simulink model "F16ASYM_Controlled_AoA"  (R2012b)
settings: Solver=ode3  SolverMode=SingleTasking  StartTime=0.0  StopTime=inf  FixedStep=T_sim  RelTol=1e-3
InitFcn:
  | load('NN_c_weights_Last_stable.mat')
values from neighbouring files (symbols this model uses):
  K_b_AoA = params(3)    [Cost_function.m]
  K_b_q = params(4)    [Cost_function.m]
  learning = 20    [Scheduling_desing.m]
  Model_used_flag = 1    [Scheduling_desing.m]
  reg_param = 0.5    [Scheduling_desing.m]
  T_sim = 0.02    [Scheduling_desing.m]
  tau_AoA = params(1)    [Cost_function.m]
  tau_q = params(2)    [Cost_function.m]
  Theta_1_roll_last = [0.00183613313267 0.00115998993235 0.0006676025148 0.00194921904952 0.00134963559861 0.00034352059664 0.000447169388141 0.00146749660935 0.00110199952389 7.77922383894e-05 0.00109492833348 0.00192687590535 ... (360 elements, 30x12)]    [NN_i_weights_LAST_STABLE.mat]
  Theta_2_roll_last = [0.000469743069697 0.000355923851088 0.00180035760697 0.00191855117771 0.00118851504447 0.0013331642065 0.0013164316578 0.000643981263341 0.00176817665434 0.000113802099363 0.000426534542462 0.00113815782354 ... (620 elements, 20x31)]    [NN_i_weights_LAST_STABLE.mat]
  Theta_3_roll_last = [9.62071520568e-05 -0.000389870886846 2.08260845013e-05 0.000140787743673 -0.000917525755397 -0.0014324207578 -0.00154701573815 -0.00131544476264 -0.00101205584381 5.06515794689e-05 -0.00111443483676 -0.00143957416141 ... (21 elements, 1x21)]    [NN_i_weights_LAST_STABLE.mat]
  V_long_lastA_w_z = [0.352826086601 -0.253633004548 -0.642535042878 0.237749930435 -0.618390629538 0.858074761295 0.268211230628 -0.448715080196 -0.0406384631192 0.401147605577 0.60598427709 0.0500551915851 ... (300 elements, 30x10)]    [NN_i_weights_LAST_STABLE.mat]
  V_long_lastAoA = [0.0774300162379 0.0911421319631 0.0352371192557 0.0542170286952 0.0651171200844 0.0177112012707 0.0982957728448 0.000259994642558 0.0194724569123 0.0466321328252 0.0556687953852 0.0252668067142 ... (300 elements, 30x10)]    [NN_i_weights_LAST_STABLE.mat]
  V_roll_last = [0.0540918675943 0.0557493347212 0.0839792276608 0.0460576391794 0.0671229058124 0.100220403067 0.0722493281881 0.0648875457457 0.00447599349201 0.0607299103823 0.0488037966361 0.0176785979393 ... (360 elements, 30x12)]    [NN_i_weights_LAST_STABLE.mat]
  V_yaw_last = [0.0965149149679 0.00833616709545 0.0365734360076 0.0523944217566 0.00790252078455 0.0700053845887 0.0345164868709 0.0111568465295 0.094060639546 0.0205483560006 0.000798047494256 0.0862769385758 ... (360 elements, 30x12)]    [NN_i_weights_LAST_STABLE.mat]
  velocity = M_eval_sche(I,J)*a    [Scheduling_desing.m]
  W_long_lastA_w_z = [-0.0522913429974 0.00385484301394 -0.00465489482472 -0.0139416219936 0.00295196421483 -0.013027768541 0.00585545058915 0.00278802233571 -0.00906272782329 -0.000396112031465 0.00405849743321 0.00509668457818 ... (31 elements, 1x31)]    [NN_i_weights_LAST_STABLE.mat]
  W_long_lastAoA = [-0.0192589013922 0.00873109909713 0.00432649597332 0.0420946902441 0.0293366820194 0.0351497798191 0.0234952374236 0.0360841187718 0.0112233388211 0.030147202199 0.0369533138617 0.00218839076415 ... (31 elements, 1x31)]    [NN_i_weights_LAST_STABLE.mat]
  W_roll_last = [-0.0006515532842 0.000535485585715 0.000550946920743 0.000806030945453 0.00045976209382 0.00065557954304 0.000945902185602 0.00070191398535 0.000635215543728 4.66501377412e-05 0.000597079583757 0.000485790566765 ... (31 elements, 1x31)]    [NN_i_weights_LAST_STABLE.mat]
  W_yaw_last = [-4.34263633305e-05 8.83823048922e-05 1.65575463724e-05 3.60293102233e-05 5.19752447623e-05 7.06399280852e-06 7.02425975821e-05 3.62680255076e-05 1.29996379937e-05 8.05072914397e-05 2.39941870661e-05 2.52427840574e-06 ... (31 elements, 1x31)]    [NN_i_weights_LAST_STABLE.mat]
undefined symbols (not defined in the file or in its folder): a1, alpha_map_eval, B, beta_map_eval, C_L_0, DiscIntNeverNeededParam, fi_flag_Simulink, G_eval, H_sq, H_sq_autotrim, k_B, m_B, M_sq, M_sq_autotrim, sigbuilder_block, Stall_curve, trim_control, trim_state, trim_throttle, V_Comp_A_w_z_last, V_Comp_last, V_roll_lastMOD, W_Comp_A_w_z_last, W_Comp_last, W_roll_lastMOD
libraries: Adaptive_FaultTolerantControl x43, dspsigops x29, F16_Actuator_Library x14, simulink x8, aerolibatmos2 x7, dsparch4 x6, simulink_extras x5, aerolibtransform2 x5, qcatlib x4, dspmtrx3 x3, dspvision x2, dspsnks4 x2
(part 9 of 11)

== matlab function F16ASYM_Controlled_AoA/SI and FDI/SI and FDI: Realistic/SI/Surfaces UKF estimator ==
  data: P input; P_out output; X_ant input; Meas input; Alt input; S_l output; TAS input; AoA input; SS input; omega_b input; Control_def input; Ctrl_effectiveness input; Deltas_Aero input; S_r output; S_f output
function [P_out,S_l,S_r,S_f] = UKF_estimator(P,X_ant,Meas,Alt,TAS,AoA,SS,omega_b,Control_def,Ctrl_effectiveness,Deltas_Aero)
% Control_def includes Throttle
% Meas are angular accelerations

m = 9295.44;
x_cg = 0.3;
Jy=75673.6;
Jxz=1331.4;
Jz=85552.1;
Jx=12874.8;

Ang_accels = zeros(3,1);
coder.extrinsic('Ang_accels_Reconf_estimator');
coder.extrinsic('schol');
coder.extrinsic('chol');

% Ang_accels = Ang_accels_Reconf_estimator([Alt,TAS,AoA,SS,omega_b',Control_def',m,  X_ant'  ,x_cg,Jy,Jxz,Jz,Jx,Ctrl_effectiveness',Deltas_Aero']');
% Ang_accels
% C_l = Ang_accels(1)
% C_m = Ang_accels(2)
% C_n = Ang_accels(3)


% S_l = 27.87/2;
% S_r=S_l;
% S_f = 6.578;
% P_out = P;


%% Filter UKF
% Init parameters 
F = eye(3);
Q = 0.005*eye(3); % Noise in the process (in surfaces)
R = 20*eye(3);   % Noise in the measures of angular acceleration

% Prediction . IT is a simple linear prediction. There is not need to do it
% in any other way because the result is the SAME
    x_pred=F*X_ant;
    x_pred(1) = max(0,min(x_pred(1),27.87/2));
    x_pred(2) = max(0,min(x_pred(2),27.87/2));
    x_pred(3) = max(0,min(x_pred(3),6.578));

    P_pred = F * P * F' + Q;

% Uncested Update
    % Measurement equations.
%     Ang_accels_Reconf_estimator([Alt,TAS,AoA,SS,omega_b',Control_def',m,  X_ant'  ,x_cg,Jy,Jxz,Jz,Jx,Ctrl_effectiveness',Deltas_Aero']')

    % Weight params
    L=size(X_ant,1);
    alpha = 1;  beta = 0;   kappa = 3 - L; % Supposed as optimals
    % %                 alpha = 0.6;  beta = 1.3;   kappa = 0.9; % Optimized by me
    
    % Generate_weights
        W_s = zeros(2*L+1,1);
        W_c = zeros(2*L+1,1);
        lambda = alpha^2 * (L + kappa) - L;
        for j=1:2*L+1
            if j==1
                W_s(j) = lambda / (L + lambda);
                W_c(j) = lambda / (L + lambda) + (1 - alpha^2 + beta);
            else
                W_s(j) = 1 / (2 * (L + lambda));
                W_c(j) = W_s(j);
            end
        end
        
    % Sigma_points
            flag = 0;
            A = zeros(size(P));
            [A,flag] = chol(P);
            A = A';
            if flag>0
                A = schol(P);
            end
        X = [zeros(size(x_pred)) A -A];
        X = sqrt(L + lambda)*X + repmat(x_pred,1,size(X,2));

    % Propagation with measurement equation (Model in this case)
        gamma_z = zeros(3,size(X,2));
        gamma_z(:,1) = Ang_accels_Reconf_estimator([Alt,TAS,AoA,SS,omega_b',Control_def',m,  X(:,1)'  ,x_cg,Jy,Jxz,Jz,Jx,Ctrl_effectiveness',Deltas_Aero']');
        for i=2:size(X,2)
%             [Alt,TAS,alpha,beta,omega_b',Control_def',m,  X(:,1)'  ,x_cg,Jy,Jxz,Jz,Jx,Ctrl_effectiveness',Deltas_Aero']
            gamma_z(:,i) = Ang_accels_Reconf_estimator([Alt,TAS,AoA,SS,omega_b',Control_def',m,  X(:,i)'  ,x_cg,Jy,Jxz,Jz,Jx,Ctrl_effectiveness',Deltas_Aero']');
        end
        
    % Update
    Z = zeros(size(gamma_z,1),1);
    Pzz  = zeros(size(gamma_z,1),size(gamma_z,1));
    Pxz  = zeros(size(x_pred,1),size(gamma_z,1));
    for i=1:size(X,2)
        Z = Z + W_s(i) * gamma_z(:,i);
    end
    for i=1:size(X,2)
        Pzz = Pzz + W_c(i) * (gamma_z(:,i) - Z) * (gamma_z(:,i) - Z)';
        Pxz = Pxz + W_c(i) * (X(1:size(x_pred,1),i) - x_pred) * (gamma_z(:,i) - Z)';
    end

    Pzz = Pzz + R;
    K = Pxz / Pzz;
    x_estimate = x_pred + K * (Meas - Z);
    P_out = P_pred - K * Pzz * K';
%     x_estimate
    S_l = x_estimate(1);
    S_r = x_estimate(2);
    S_f = x_estimate(3);

== matlab function F16ASYM_Controlled_AoA/Primary Controller/P  + Crossed NN + AWU+Lim + hand-over/P controller + adaptive Crossed NN + AWU+Lim    in ACC /Complete crossed On-line (adaptive) multi-layer NN: A_w_z/Cross NN A_w_z ==
  data: X_bar input size=[25,1]; v_ad_comp output; e input; Factor_F input; K_roll input; Ks_long input; Ks_yaw input; B input; Learnign_rate input size=1; Reg_param input size=1; AWU input; W input size=[3,51]; V input size=[50,25]; v_ad output; Z_norm_unit output; T_sim parameter; W_update output; V_update output
function [v_ad_comp,v_ad,Z_norm_unit,W_update,V_update]  = Cross_NN(X_bar,e,Factor_F, K_roll,Ks_long,Ks_yaw,B,Learnign_rate,Reg_param,AWU,W,V,T_sim)

%% Compute prelimiary parametes
% Compute P with regular Lyapunov equation solution
P_roll=1/K_roll;
P_long =  [   1/Ks_long(1) , Factor_F/(Ks_long(1)^2+Ks_long(1)*Ks_long(2));
     1/(Ks_long(1)^2+Ks_long(1)*Ks_long(2)) ,(Ks_long(1)^2+Ks_long(1)*Ks_long(2)+Factor_F^2)/(Ks_long(2)^2*Ks_long(1)+Ks_long(2)*Ks_long(1)^2) ];
P_yaw = [   1/Ks_yaw(1) , 1/(Ks_yaw(1)^2+Ks_yaw(1)*Ks_yaw(2));
     1/(Ks_yaw(1)^2+Ks_yaw(1)*Ks_yaw(2)) ,(Ks_yaw(1)^2+Ks_yaw(1)*Ks_yaw(2)+1)/(Ks_yaw(2)^2*Ks_yaw(1)+Ks_yaw(2)*Ks_yaw(1)^2) ];
 
P = blkdiag(P_roll,P_long,P_yaw);

% % % % Compute P with on-line Lyapunov equation solution
% % % CROSS = 0;
% % % A = [ -K_roll,0,CROSS,0,0;0,-Ks_long(1),1,0,0;
% % %     0,0,-Ks_long(2),0,0;0,0,0,-Ks_yaw(1),Factor_F;0,0,0,0,-Ks_yaw(2)];
% % % 
% % % coder.extrinsic('lyap')
% % % P = A;
% % % P = lyap(A,2*diag(ones(5,1)));



K_awu = 1.2;
zeta= e'*P*B;


% Introduce Anti-windup
zeta = zeta - K_awu*AWU'.*T_sim; 

% Convergence limitation
if norm(zeta)>2/(T_sim*Learnign_rate*Reg_param)
    zeta = (zeta./norm(zeta)).*(1.8/(T_sim*Learnign_rate*Reg_param));
end

%% Feedforward
z = V*X_bar;
s=sigmoid(V*X_bar);

sigma = [1 ; s ];
% v_ad = W*sigma;

sigma_grad = (sigma.*(ones(size(sigma))-sigma));

%% Compute the gradients or adaptation laws
Gamma_w= Learnign_rate; % W learnign rate
Gamma_v= Learnign_rate; %V learning rate
lambda = Reg_param;

V_dot=zeros(size(V));
W_dot=zeros(size(W));

W_dot= -Gamma_w*(  (sigma - sigma_grad.*[1;z] )*zeta  )';
W_dot(:,2:end)= W_dot(:,2:end) - Gamma_w*lambda*norm(zeta)*(W(:,2:end));

M = W'*zeta'.*sigma_grad ;
V_dot= -Gamma_v*( M(2:end)*X_bar'  );
V_dot(:,2:end)= V_dot(:,2:end) - Gamma_v*lambda*norm(zeta).*V(:,2:end);

% % % Other way: Based on notes of Andrew NG
% % 
% % delta2=W'*zeta'.*sigma_grad;
% % 
% % V_dot = - Gamma_v*( delta2(2:end)*X_bar');
% % V_dot(:,2:end)= V_dot(:,2:end) - Gamma_v*lambda*norm(zeta).*V(:,2:end);
% % 
% % W_dot = - Gamma_w*( sigma*zeta)';
% % W_dot(:,2:end)= W_dot(:,2:end) - Gamma_w*lambda*norm(zeta)*(W(:,2:end));



%% Adaptation
W_update = W + T_sim*W_dot;
V_update = V + T_sim*V_dot;
% 
%% Re-compute v_ad

s=sigmoid(V_update*X_bar);

sigma = [1 ; s(:,1) ];
v_ad = W_update*sigma;

%% Compute v_ad_comp
Z = [ V,zeros(size(V,1),size(W,2));
    zeros(size(W,1),size(V,2)),W];
    
Z_norm = norm(Z,'fro');
Z_max = 2*min(size(W,1),size(W,2) )*min( size(V,1),size(V,2) );
Z_norm_unit = Z_norm;

K_r0= 0;
K_r1= 0;
v_r0 = -K_r0*zeta';
v_r1 = -K_r1*(Z_norm+Z_max)*zeta';

v_ad_comp = v_ad + v_r1 +v_r0;

% % % Normalization of matrices
% % if Z_norm>Z_max
% %     V = (V.*Z_max)./Z_norm;
% %     W = (W.*Z_max)./Z_norm;
% % end
end

== system F16ASYM_Controlled_AoA/Primary Controller/P controller + adaptive Crossed NN + AWU+Lim /Complete crossed On-line (adaptive) multi-layer NN/Complete crossed On-line (adaptive) multi-layer NN: AoA ==
  v_ad^ prev : Inport
  All_meas : Inport  Port=2
  NN variables : Inport  Port=3
  AWU : Inport  Port=4
  B : Constant  Value=[1 0 0;0 0 0;0 1 0;0 0 0;0 0 1]
  Bus Selector : BusSelector  OutputSignals=p_chanel_vars,Long chanel,beta_r_chanel
  Bus Selector1 : BusSelector  OutputSignals=p_err,p_sf,p_sf_dot,K_b_p
  Bus Selector2 : BusSelector  OutputSignals=signal1.Alt meas (m),signal2.Mach,signal1.AoA meas (rad),signal1.SS meas (rad),signal1.omega_b meas (rad/s)
  Bus Selector3 : BusSelector  OutputSignals=alpha_chanel vars.alpha_err,q_chanel_vars.q_err,alpha_chanel vars.alpha_sf,alpha_chanel vars.alpha_sf_dot,q_chanel_vars.q_sf_dot,alpha_chanel vars.K_b_alpha,q_chanel_vars.K_b_q
  Bus Selector4 : BusSelector  OutputSignals=beta_chanel vars.beta_err,r_chanel vars.r_err,beta_chanel vars.beta_sf,beta_chanel vars.beta_sf_dot,r_chanel vars.r_sf_dot,beta_chanel vars.K_b_beta,r_chanel vars.K_b_r
  C Learning rate : Constant  Value=30  SampleTime=T_sim
  C Reg param : Constant  Value=0.5  SampleTime=T_sim
  Constant : Constant
  Cross NN : MATLAB Function  TreatAsAtomicUnit=on
  Display : Display
  Divide : Product  Inputs=**
  Divide1 : Product  Inputs=**
  Memory2 : Memory  X0=V_Comp_last
  Memory3 : Memory  X0=W_Comp_last
  Mux1 : Mux  Inputs=9
  Mux10 : Mux  Inputs=3
  Mux2 : Mux  Inputs=3
  Mux{3..4,6..7} (4 alike) : Mux  Inputs=2
  Mux5 : Mux  Inputs=5
  Mux8 : Mux  Inputs=5
  Mux9 : Mux  Inputs=[9 3 5 5 3]
  Scope : Scope
      settings: SaveName=ScopeData8
  Selector : Selector  InputPortWidth=3  IndexOptions=Index vector (dialog)  Indices=1  OutputSizes=1
  Selector1 : Selector  InputPortWidth=3  IndexOptions=Index vector (dialog)  Indices=3  OutputSizes=1
  Terminator : Terminator
  Terminator1 : Terminator
  To Workspace : ToWorkspace  VariableName=V_Comp_last  SampleTime=-1
      settings: MaxDataPoints=1
  To Workspace1 : ToWorkspace  VariableName=W_Comp_last  SampleTime=-1
      settings: MaxDataPoints=1
  dem-less : Gain  Gain=T_sim
  dem-less1 : Gain  Gain=T_sim
  dem-less2 : Gain  Gain=T_sim^2
  dem-less3 : Gain  Gain=T_sim
  dem-less4 : Gain  Gain=T_sim^2
  dim-less : Gain  Gain=1/15000
  v_ad^ : Outport
  wires:
  Bus Selector/3 -> Bus Selector4/1  "<beta_r_chanel>"
  Bus Selector/2 -> Bus Selector3/1  "<Long chanel>"
  Bus Selector/1 -> Bus Selector1/1  "<p_chanel_vars>"
  NN variables/1 -> Bus Selector/1
  Bus Selector2/5 -> Selector1/1, Selector/1  "<omega_b meas (rad/s)>"
  dim-less/1 -> Mux1/2
  Divide1/1 -> Mux1/6
  Divide/1 -> Mux1/4
  Bus Selector2/1 -> dim-less/1  "<Alt meas (m)>"
  All_meas/1 -> Bus Selector2/1
  Constant/1 -> Mux1/1
  Bus Selector1/3 -> dem-less/1  "<p_sf_dot>"
  Selector/1 -> Mux1/8
  Bus Selector2/4 -> Mux1/7  "<SS meas (rad)>"
  Bus Selector2/2 -> Divide/2, Mux1/3, Divide/1  "<Mach>"
  Bus Selector2/3 -> Divide1/1, Mux1/5, Divide1/2  "<AoA meas (rad)>"
  Bus Selector1/4 -> [K_roll]  "<K_b_p>"
  Bus Selector1/2 -> Mux2/2  "<p_sf>"
  Bus Selector1/1 -> [e_roll], Mux2/1  "<p_err>"
  dem-less/1 -> Mux2/3
  dem-less2/1 -> Mux5/5
  dem-less1/1 -> Mux5/4
  Mux4/1 -> [Ks_long]
  Bus Selector3/6 -> Mux4/1  "<K_b_alpha>"
  Bus Selector3/7 -> Mux4/2  "<K_b_q>"
  Bus Selector3/5 -> dem-less2/1  "<q_sf_dot>"
  Bus Selector3/4 -> dem-less1/1  "<alpha_sf_dot>"
  Bus Selector3/1 -> Mux5/1, Mux3/1  "<alpha_err>"
  Bus Selector3/2 -> Mux5/2, Mux3/2  "<q_err>"
  Bus Selector3/3 -> Mux5/3  "<alpha_sf>"
  Mux3/1 -> [e_long]  "e"
  dem-less3/1 -> Mux8/4
  Bus Selector4/3 -> Mux8/3  "<beta_sf>"
  Bus Selector4/4 -> dem-less3/1  "<beta_sf_dot>"
  Bus Selector4/5 -> dem-less4/1  "<r_sf_dot>"
  Bus Selector4/7 -> Mux6/2  "<K_b_r>"
  Bus Selector4/6 -> Mux6/1  "<K_b_beta>"
  Mux6/1 -> [Ks_yaw]
  Bus Selector4/1 -> Mux8/1, Mux7/1  "<beta_err>"
  Bus Selector4/2 -> Mux8/2, Mux7/2  "<r_err>"
  Mux7/1 -> [e_yaw]  "e"
  dem-less4/1 -> Mux8/5
  Mux1/1 -> Mux9/1
  Mux2/1 -> Mux9/2
  Mux5/1 -> Mux9/3
  Mux8/1 -> Mux9/4
  v_ad^ prev/1 -> Mux9/5
  Mux9/1 -> Scope/1, Display/1, Cross NN/1(X_bar)
  Cross NN/3(Z_norm_unit) -> Terminator1/1
  C Reg param/1 -> Cross NN/8(Reg_param)
  C Learning rate/1 -> Cross NN/7(Learnign_rate)
  Cross NN/1(v_ad_comp) -> v_ad^/1
  Memory2/1 -> Cross NN/11(V)
  Memory3/1 -> Cross NN/10(W)
  B/1 -> Cross NN/6(B)
  Cross NN/2(v_ad) -> Terminator/1
  Cross NN/5(V_update) -> To Workspace/1, Memory2/1
  Cross NN/4(W_update) -> Memory3/1, To Workspace1/1
  Mux10/1 -> Cross NN/2(e)
  [e_roll] -> Mux10/1
  [e_long] -> Mux10/2
  [e_yaw] -> Mux10/3
  [K_roll] -> Cross NN/3(K_roll)
  [Ks_long] -> Cross NN/4(Ks_long)
  [Ks_yaw] -> Cross NN/5(Ks_yaw)
  Selector1/1 -> Mux1/9
  AWU/1 -> Cross NN/9(AWU)

== system F16ASYM_Controlled_AoA/Primary Controller/P controller + adaptive Crossed NN + AWU+Lim /Long Dyn Inversion: alpha_dot ->q/Completed ==
  alpha_dot_c : Inport
  All_meas : Inport  Port=2
  A_w_z : Selector  InputPortWidth=3  IndexOptions=Index vector (dialog)  Indices=3  OutputSizes=1
  Add : Sum
  Bus Selector : BusSelector  OutputSignals=signal1.AoA meas (rad),signal1.omega_b meas (rad/s),signal1.SS meas (rad),signal1.V_TAS (m/s),signal2.A_w_CG
  Display : Display
  Display1 : Display
  Display2 : Display
  Divide{,1..3} (4 alike) : Product  Inputs=**
  Divide4 : Product  Inputs=/*
  Selector : Selector  InputPortWidth=3  IndexOptions=Index vector (dialog)  Indices=1  OutputSizes=1
  Selector1 : Selector  InputPortWidth=3  IndexOptions=Index vector (dialog)  Indices=3  OutputSizes=1
  Trigonometric Function : Trigonometry  Operator=sincos
  Trigonometric Function1 : Trigonometry  Operator=tan
  Trigonometric Function2 : Trigonometry  Operator=cos
  "q_c " : Sum  Inputs=++-
  q_c : Outport
  wires:
  Trigonometric Function/1 -> Divide1/1
  Bus Selector/1 -> Trigonometric Function/1  "<AoA meas (rad)>"
  Selector/1 -> Divide/2
  Bus Selector/2 -> Selector1/1, Selector/1  "<omega_b meas (rad/s)>"
  Divide2/1 -> "q_c "/2, Display1/1
  Selector1/1 -> Divide1/2
  Divide3/1 -> Divide4/1
  alpha_dot_c/1 -> "q_c "/1, Display/1
  All_meas/1 -> Bus Selector/1
  Bus Selector/5 -> A_w_z/1  "<A_w_CG>"
  Bus Selector/3 -> Trigonometric Function1/1, Trigonometric Function2/1  "<SS meas (rad)>"
  Divide4/1 -> "q_c "/3
  "q_c "/1 -> q_c/1
  Divide/1 -> Add/1
  Bus Selector/4 -> Divide3/2  "<V_TAS (m/s)>"
  Add/1 -> Divide2/1
  Trigonometric Function1/1 -> Divide2/2
  Divide1/1 -> Add/2
  Trigonometric Function2/1 -> Divide3/1
  Trigonometric Function/2 -> Divide/1
  A_w_z/1 -> Display2/1, Divide4/2

== system F16ASYM_Controlled_AoA/Primary Controller/P controller + adaptive Crossed NN + AWU+Lim /Long Dyn Inversion: alpha_dot ->q/Simplified ==
  alpha_dot_c : Inport
  All_meas : Inport  Port=2
  A_b_z : Selector  InputPortWidth=3  IndexOptions=Index vector (dialog)  Indices=3  OutputSizes=1
  Bus Selector : BusSelector  OutputSignals=signal2.A_b_CG,signal1.V_TAS (m/s)
  Display : Display
  Divide4 : Product  Inputs=*/
  "q_c " : Sum  Inputs=+-
  q_c : Outport
  wires:
  "q_c "/1 -> q_c/1
  All_meas/1 -> Bus Selector/1
  alpha_dot_c/1 -> "q_c "/1, Display/1
  Bus Selector/2 -> Divide4/2  "<V_TAS (m/s)>"
  Divide4/1 -> "q_c "/2
  A_b_z/1 -> Divide4/1  "A_b_z"
  Bus Selector/1 -> A_b_z/1  "<A_b_CG>"

== system F16ASYM_Controlled_AoA/Primary Controller/P controller + adaptive Crossed NN + AWU+Lim /Longitudinal Controller: AoA or A_w_z/Longitudinal controller in A_w_z ==
  A_w_z des : Inport
  AoA des (rad) : Inport  Port=2
  Anti-windup A_w_z : Inport  Port=3
  Anti-windup AoA : Inport  Port=4
  All meas : Inport  Port=5
  Accel rate --> AoA rate! : Subsystem
  Bus Creator : BusCreator  Inputs=5
  Bus Selector : BusSelector  OutputSignals=signal2.A_w_CG
  Divide : Product  Inputs=**
  Gain : Gain  Gain=-1
  Ground : Ground
  Ref Model and P Controller : Adaptive_FaultTolerantControl/Ref Model and P Controller  tau=0.3  y_i=0  K_f=1  K_b=2.5
  Selector : Selector  InputPortWidth=3  IndexOptions=Index vector (dialog)  Indices=3  OutputSizes=1
  Stall protection : Subsystem  Commented=on
  Sum : Sum  Inputs=+-|
  Terminator : Terminator
  Terminator1 : Terminator
  Terminator2 : Terminator
  A_chanel vars : Outport
  alpha_chanel vars : Outport  Port=2
  alpha_dot_c : Outport  Port=3
  wires:
  Anti-windup AoA/1 -> Terminator1/1
  AoA des (rad)/1 -> Terminator/1
  Selector/1 -> Gain/1
  Gain/1 -> Ref Model and P Controller/2
  Bus Selector/1 -> Selector/1  "<A_w_CG>"
  Anti-windup A_w_z/1 -> Terminator2/1
  A_w_z des/1 -> Ref Model and P Controller/1
  Ref Model and P Controller/1 -> Divide/1
  Ref Model and P Controller/2 -> Bus Creator/1  "A_sf_dot"
  Ref Model and P Controller/3 -> Bus Creator/2, Sum/1  "A_sf"
  Sum/1 -> Bus Creator/3  "A_err"
  Ref Model and P Controller/4 -> Sum/2
  Ref Model and P Controller/5 -> Bus Creator/4  "K_b_A"
  Bus Creator/1 -> A_chanel vars/1
  Ground/1 -> alpha_chanel vars/1
  Divide/1 -> alpha_dot_c/1
  Accel rate --> AoA rate!/1(A_w  to AoA rates factor) -> Bus Creator/5, Divide/2  "FactorF"
  All meas/1 -> Bus Selector/1, Stall protection/2(All meas), Accel rate --> AoA rate!/1(All_meas)

== system F16ASYM_Controlled_AoA/Primary Controller/P controller + adaptive Crossed NN + AWU+Lim /Longitudinal Controller: AoA or A_w_z/Longitudinal controller in AoA ==
  A_w_z des : Inport
  AoA des (rad) : Inport  Port=2
  Anti-windup A_w_z : Inport  Port=3
  Anti-windup AoA : Inport  Port=4
  All meas : Inport  Port=5
  Bus Creator : BusCreator
  Bus Selector : BusSelector  OutputSignals=signal1.AoA meas (rad)
  Ground : Ground
  Ref Model and P Controller : Adaptive_FaultTolerantControl/Ref Model and P Controller  tau=0.3  y_i=trim_state(8)  K_f=1  K_b=8
  Sum : Sum  Inputs=+-|
  Terminator : Terminator
  Terminator1 : Terminator
  Terminator2 : Terminator
  A_chanel vars : Outport
  alpha_chanel vars : Outport  Port=2
  alpha_dot_c : Outport  Port=3
  wires:
  All meas/1 -> Bus Selector/1
  Ref Model and P Controller/1 -> alpha_dot_c/1
  Bus Selector/1 -> Ref Model and P Controller/2  "<AoA meas (rad)>"
  AoA des (rad)/1 -> Ref Model and P Controller/1
  A_w_z des/1 -> Terminator/1
  Anti-windup A_w_z/1 -> Terminator1/1
  Anti-windup AoA/1 -> Terminator2/1
  Ref Model and P Controller/2 -> Bus Creator/1  "alpha_sf_dot"
  Ref Model and P Controller/3 -> Sum/1, Bus Creator/2  "alpha_sf"
  Sum/1 -> Bus Creator/3  "alpha_err"
  Bus Creator/1 -> alpha_chanel vars/1
  Ref Model and P Controller/4 -> Sum/2
  Ref Model and P Controller/5 -> Bus Creator/4  "K_b_alpha"
  Ground/1 -> A_chanel vars/1

== system F16ASYM_Controlled_AoA/Primary Controller/P controller + adaptive Crossed NN + AWU+Lim /Physical limitation/Moments ==
  C_L : Inport
  C_M : Inport  Port=2
  C_N : Inport  Port=3
  q : Inport  Port=4
  B span : Constant  Value=9.144
  CMA : Constant  Value=3.45
  Divide : Product  Inputs=**
  Divide1 : Product  Inputs=***
  Divide2 : Product  Inputs=**
  Divide3 : Product  Inputs=***
  Divide4 : Product  Inputs=**
  S_w : Constant  Value=27.87
  S_w1 : Constant  Value=27.87
  q1 : InportShadow  Port=4
  L : Outport
  M : Outport  Port=2
  N : Outport  Port=3
  wires:
  Divide4/1 -> M/1  "M"
  Divide3/1 -> Divide4/2
  C_M/1 -> Divide4/1
  CMA/1 -> Divide3/3
  S_w1/1 -> Divide3/2
  q1/1 -> Divide3/1
  Divide2/1 -> N/1  "N"
  C_N/1 -> Divide2/2
  Divide/1 -> L/1  "L"
  Divide1/1 -> Divide/2, Divide2/1
  C_L/1 -> Divide/1
  B span/1 -> Divide1/3
  S_w/1 -> Divide1/2
  q/1 -> Divide1/1

== system F16ASYM_Controlled_AoA/Primary Controller/P controller + adaptive Isolated NN/Long Dyn Inversion: alpha_dot ->q/Completed ==
  alpha_dot_c : Inport
  All_meas : Inport  Port=2
  A_w_z : Selector  InputPortWidth=3  IndexOptions=Index vector (dialog)  Indices=3  OutputSizes=1
  Add : Sum
  Bus Selector : BusSelector  OutputSignals=signal1.AoA meas (rad),signal1.omega_b meas (rad/s),signal1.SS meas (rad),signal1.V_TAS (m/s),signal2.A_w_CG
  Display : Display
  Display1 : Display
  Display2 : Display
  Divide{,1..3} (4 alike) : Product  Inputs=**
  Divide4 : Product  Inputs=/*
  Selector : Selector  InputPortWidth=3  IndexOptions=Index vector (dialog)  Indices=1  OutputSizes=1
  Selector1 : Selector  InputPortWidth=3  IndexOptions=Index vector (dialog)  Indices=3  OutputSizes=1
  Trigonometric Function : Trigonometry  Operator=sincos
  Trigonometric Function1 : Trigonometry  Operator=tan
  Trigonometric Function2 : Trigonometry  Operator=cos
  "q_c " : Sum  Inputs=++-
  q_c : Outport
  wires:
  Trigonometric Function/1 -> Divide1/1
  Bus Selector/1 -> Trigonometric Function/1  "<AoA meas (rad)>"
  Selector/1 -> Divide/2
  Bus Selector/2 -> Selector1/1, Selector/1  "<omega_b meas (rad/s)>"
  Divide2/1 -> "q_c "/2, Display1/1
  Selector1/1 -> Divide1/2
  Divide3/1 -> Divide4/1
  alpha_dot_c/1 -> "q_c "/1, Display/1
  All_meas/1 -> Bus Selector/1
  Bus Selector/5 -> A_w_z/1  "<A_w_CG>"
  Bus Selector/3 -> Trigonometric Function1/1, Trigonometric Function2/1  "<SS meas (rad)>"
  Divide4/1 -> "q_c "/3
  "q_c "/1 -> q_c/1
  Divide/1 -> Add/1
  Bus Selector/4 -> Divide3/2  "<V_TAS (m/s)>"
  Add/1 -> Divide2/1
  Trigonometric Function1/1 -> Divide2/2
  Divide1/1 -> Add/2
  Trigonometric Function2/1 -> Divide3/1
  Trigonometric Function/2 -> Divide/1
  A_w_z/1 -> Display2/1, Divide4/2

== system F16ASYM_Controlled_AoA/Primary Controller/P controller + adaptive Isolated NN/Long Dyn Inversion: alpha_dot ->q/Simplified ==
  alpha_dot_c : Inport
  All_meas : Inport  Port=2
  A_b_z : Selector  InputPortWidth=3  IndexOptions=Index vector (dialog)  Indices=3  OutputSizes=1
  Bus Selector : BusSelector  OutputSignals=signal2.A_b_CG,signal1.V_TAS (m/s)
  Display : Display
  Divide4 : Product  Inputs=*/
  "q_c " : Sum  Inputs=+-
  q_c : Outport
  wires:
  "q_c "/1 -> q_c/1
  All_meas/1 -> Bus Selector/1
  alpha_dot_c/1 -> "q_c "/1, Display/1
  Bus Selector/2 -> Divide4/2  "<V_TAS (m/s)>"
  Divide4/1 -> "q_c "/2
  A_b_z/1 -> Divide4/1  "A_b_z"
  Bus Selector/1 -> A_b_z/1  "<A_b_CG>"

== system F16ASYM_Controlled_AoA/Primary Controller/P controller + adaptive Isolated NN/Longitudinal Controller: AoA or A_w_z/Longitudinal controller in A_w_z ==
  A_w_z des : Inport
  AoA des (rad) : Inport  Port=2
  Anti-windup A_w_z : Inport  Port=3
  Anti-windup AoA : Inport  Port=4
  All meas : Inport  Port=5
  Accel rate --> AoA rate! : Subsystem
  Bus Creator : BusCreator  Inputs=5
  Bus Selector : BusSelector  OutputSignals=signal2.A_w_CG
  Divide : Product  Inputs=**
  Gain : Gain  Gain=-1
  Ground : Ground
  Ref Model and P Controller : Adaptive_FaultTolerantControl/Ref Model and P Controller  tau=0.1  y_i=0  K_f=1  K_b=3.1
  Selector : Selector  InputPortWidth=3  IndexOptions=Index vector (dialog)  Indices=3  OutputSizes=1
  Sum : Sum  Inputs=+-|
  Terminator : Terminator
  Terminator1 : Terminator
  Terminator2 : Terminator
  A_chanel vars : Outport
  alpha_chanel vars : Outport  Port=2
  alpha_dot_c : Outport  Port=3
  wires:
  Anti-windup AoA/1 -> Terminator1/1
  AoA des (rad)/1 -> Terminator/1
  Selector/1 -> Gain/1
  Gain/1 -> Ref Model and P Controller/2
  Bus Selector/1 -> Selector/1  "<A_w_CG>"
  All meas/1 -> Bus Selector/1, Accel rate --> AoA rate!/1(All_meas)
  Anti-windup A_w_z/1 -> Terminator2/1
  A_w_z des/1 -> Ref Model and P Controller/1
  Ref Model and P Controller/1 -> Divide/1
  Ref Model and P Controller/2 -> Bus Creator/1  "A_sf_dot"
  Ref Model and P Controller/3 -> Bus Creator/2, Sum/1  "A_sf"
  Sum/1 -> Bus Creator/3  "A_err"
  Ref Model and P Controller/4 -> Sum/2
  Ref Model and P Controller/5 -> Bus Creator/4  "K_b_A"
  Bus Creator/1 -> A_chanel vars/1
  Ground/1 -> alpha_chanel vars/1
  Divide/1 -> alpha_dot_c/1
  Accel rate --> AoA rate!/1(A_w  to AoA rates factor) -> Bus Creator/5, Divide/2  "FactorF"

== system F16ASYM_Controlled_AoA/Primary Controller/P controller + adaptive Isolated NN/Longitudinal Controller: AoA or A_w_z/Longitudinal controller in AoA ==
  A_w_z des : Inport
  AoA des (rad) : Inport  Port=2
  Anti-windup A_w_z : Inport  Port=3
  Anti-windup AoA : Inport  Port=4
  All meas : Inport  Port=5
  Bus Creator : BusCreator
  Bus Selector : BusSelector  OutputSignals=signal1.AoA meas (rad)
  Ground : Ground
  Ref Model and P Controller : Adaptive_FaultTolerantControl/Ref Model and P Controller  tau=0.3  y_i=trim_state(8)  K_f=1  K_b=8
  Sum : Sum  Inputs=+-|
  Terminator : Terminator
  Terminator1 : Terminator
  Terminator2 : Terminator
  A_chanel vars : Outport
  alpha_chanel vars : Outport  Port=2
  alpha_dot_c : Outport  Port=3
  wires:
  All meas/1 -> Bus Selector/1
  Ref Model and P Controller/1 -> alpha_dot_c/1
  Bus Selector/1 -> Ref Model and P Controller/2  "<AoA meas (rad)>"
  AoA des (rad)/1 -> Ref Model and P Controller/1
  A_w_z des/1 -> Terminator/1
  Anti-windup A_w_z/1 -> Terminator1/1
  Anti-windup AoA/1 -> Terminator2/1
  Ref Model and P Controller/2 -> Bus Creator/1  "alpha_sf_dot"
  Ref Model and P Controller/3 -> Sum/1, Bus Creator/2  "alpha_sf"
  Sum/1 -> Bus Creator/3  "alpha_err"
  Bus Creator/1 -> alpha_chanel vars/1
  Ref Model and P Controller/4 -> Sum/2
  Ref Model and P Controller/5 -> Bus Creator/4  "K_b_alpha"
  Ground/1 -> A_chanel vars/1

== system F16ASYM_Controlled_AoA/Primary Controller/P controller + adaptive Isolated NN/On-line (adaptive) multi-layer NNs/Long Chanel ==
  v_ad^ prev : Inport
  Long_chanel vars : Inport  Port=2
  All_meas : Inport  Port=3
  Long_learning rate : Inport  Port=4
  Long reg param : Inport  Port=5
  Long HL NN A_w_z : Subsystem  VariantObject=Long HL NN A_w_z
  Long HL NN AoA : Subsystem  VariantObject=Long HL NN AoA
  v_ad_comp : Outport

== system F16ASYM_Controlled_AoA/Primary Controller/P controller + adaptive Isolated NN/On-line (adaptive) multi-layer NNs/Roll NN ==
  v_ad^ prev : Inport
  p_chanel vars : Inport  Port=2
  All_meas : Inport  Port=3
  Roll_learning rate : Inport  Port=4
  Roll reg param : Inport  Port=5
  Roll 1HL NN : Subsystem  VariantObject=Roll 1HL NN
  Roll 2HL NN : Subsystem  VariantObject=Roll 2HL NN
  v_ad_comp : Outport

== system F16ASYM_Controlled_AoA/Primary Controller/P controller + adaptive Isolated NN/On-line (adaptive) multi-layer NNs/Yaw Chanel ==
  v_ad^ prev : Inport
  Yaw_chanel vars : Inport  Port=2
  All_meas : Inport  Port=3
  Yaw_learning rate : Inport  Port=4
  Yaw reg param : Inport  Port=5
  Yaw HL NN : Subsystem  VariantObject=Yaw HL NN
  v_ad_comp : Outport

== system F16ASYM_Controlled_AoA/Primary Controller/P controller + adaptive Isolated NN/On-line (adaptive) multi-layer NNs SIMPL/Long Chanel ==
  v_ad^ prev : Inport
  Long_chanel vars : Inport  Port=2
  All_meas : Inport  Port=3
  Long_learning rate : Inport  Port=4
  Long reg param : Inport  Port=5
  Long HL NN A_w_z : Subsystem  VariantObject=Long HL NN A_w_z
  Long HL NN AoA : Subsystem  VariantObject=Long HL NN AoA
  v_ad_comp : Outport

== system F16ASYM_Controlled_AoA/Primary Controller/P controller + adaptive Isolated NN/On-line (adaptive) multi-layer NNs SIMPL/Roll NN ==
  v_ad^ prev : Inport
  p_chanel vars : Inport  Port=2
  All_meas : Inport  Port=3
  Roll_learning rate : Inport  Port=4
  Roll reg param : Inport  Port=5
  Roll 1HL NN : Subsystem  VariantObject=Roll 1HL NN
  Roll 2HL NN : Subsystem  VariantObject=Roll 2HL NN
  v_ad_comp : Outport

== system F16ASYM_Controlled_AoA/Primary Controller/P controller + adaptive Isolated NN/On-line (adaptive) multi-layer NNs SIMPL/Yaw Chanel ==
  v_ad^ prev : Inport
  Yaw_chanel vars : Inport  Port=2
  All_meas : Inport  Port=3
  Yaw_learning rate : Inport  Port=4
  Yaw reg param : Inport  Port=5
  Yaw HL NN : Subsystem  VariantObject=Yaw HL NN
  v_ad_comp : Outport

== system F16ASYM_Controlled_AoA/Primary Controller/PI Primary Controller/Long Dyn Inversion: alpha_dot ->q/Completed ==
  alpha_dot_c : Inport
  All_meas : Inport  Port=2
  A_w_z : Selector  InputPortWidth=3  IndexOptions=Index vector (dialog)  Indices=3  OutputSizes=1
  Add : Sum
  Bus Selector : BusSelector  OutputSignals=signal1.AoA meas (rad),signal1.omega_b meas (rad/s),signal1.SS meas (rad),signal1.V_TAS (m/s),signal2.A_w_CG
  Display : Display
  Display1 : Display
  Display2 : Display
  Divide{,1..3} (4 alike) : Product  Inputs=**
  Divide4 : Product  Inputs=/*
  Selector : Selector  InputPortWidth=3  IndexOptions=Index vector (dialog)  Indices=1  OutputSizes=1
  Selector1 : Selector  InputPortWidth=3  IndexOptions=Index vector (dialog)  Indices=3  OutputSizes=1
  Trigonometric Function : Trigonometry  Operator=sincos
  Trigonometric Function1 : Trigonometry  Operator=tan
  Trigonometric Function2 : Trigonometry  Operator=cos
  "q_c " : Sum  Inputs=++-
  q_c : Outport
  wires:
  A_w_z/1 -> Divide4/2, Display2/1
  Trigonometric Function/2 -> Divide/1
  Trigonometric Function2/1 -> Divide3/1
  Divide1/1 -> Add/2
  Trigonometric Function1/1 -> Divide2/2
  Add/1 -> Divide2/1
  Bus Selector/4 -> Divide3/2  "<V_TAS (m/s)>"
  Divide/1 -> Add/1
  "q_c "/1 -> q_c/1
  Divide4/1 -> "q_c "/3
  Bus Selector/3 -> Trigonometric Function2/1, Trigonometric Function1/1  "<SS meas (rad)>"
  Bus Selector/5 -> A_w_z/1  "<A_w_CG>"
  All_meas/1 -> Bus Selector/1
  alpha_dot_c/1 -> Display/1, "q_c "/1
  Divide3/1 -> Divide4/1
  Selector1/1 -> Divide1/2
  Divide2/1 -> Display1/1, "q_c "/2
  Bus Selector/2 -> Selector/1, Selector1/1  "<omega_b meas (rad/s)>"
  Selector/1 -> Divide/2
  Bus Selector/1 -> Trigonometric Function/1  "<AoA meas (rad)>"
  Trigonometric Function/1 -> Divide1/1

== system F16ASYM_Controlled_AoA/Primary Controller/PI Primary Controller/Long Dyn Inversion: alpha_dot ->q/Simplified ==
  alpha_dot_c : Inport
  All_meas : Inport  Port=2
  A_b_z : Selector  InputPortWidth=3  IndexOptions=Index vector (dialog)  Indices=3  OutputSizes=1
  Bus Selector : BusSelector  OutputSignals=signal2.A_b_CG,signal1.V_TAS (m/s)
  Display : Display
  Divide4 : Product  Inputs=*/
  "q_c " : Sum  Inputs=+-
  q_c : Outport
  wires:
  Bus Selector/1 -> A_b_z/1  "<A_b_CG>"
  A_b_z/1 -> Divide4/1  "A_b_z"
  Divide4/1 -> "q_c "/2
  Bus Selector/2 -> Divide4/2  "<V_TAS (m/s)>"
  alpha_dot_c/1 -> Display/1, "q_c "/1
  All_meas/1 -> Bus Selector/1
  "q_c "/1 -> q_c/1

== system F16ASYM_Controlled_AoA/Primary Controller/PI Primary Controller/Longitudinal Controller: AoA or A_w_z/Longitudinal controller in A_w_z ==
  A_w_z des : Inport
  AoA des (rad) : Inport  Port=2
  Anti-windup A_w_z : Inport  Port=3
  Anti-windup AoA : Inport  Port=4
  All meas : Inport  Port=5
  Accel rate --> AoA rate! : Subsystem
  Bus Selector : BusSelector  OutputSignals=signal2.A_w_CG
  Gain : Gain  Gain=-1
  PI Controller: A_w_z  controller : Adaptive_FaultTolerantControl/PI Controller  delta=0  K_a=0  y_i=0  Des_way=pro  omega_n=2  xi=0.8  Z1=-40  K_b=2  f_i=0.5  f_c=1
  Selector : Selector  InputPortWidth=3  IndexOptions=Index vector (dialog)  Indices=3  OutputSizes=1
  Terminator : Terminator
  Terminator1 : Terminator
  alpha_dot_c : Outport
  wires:
  PI Controller: A_w_z  controller/1 -> Accel rate --> AoA rate!/1(A_w_z dot)
  A_w_z des/1 -> PI Controller: A_w_z  controller/1
  Anti-windup A_w_z/1 -> PI Controller: A_w_z  controller/3
  All meas/1 -> Accel rate --> AoA rate!/2(All_meas), Bus Selector/1
  Bus Selector/1 -> Selector/1  "<A_w_CG>"
  Accel rate --> AoA rate!/1(alpha_dot des) -> alpha_dot_c/1
  Gain/1 -> PI Controller: A_w_z  controller/2
  Selector/1 -> Gain/1
  AoA des (rad)/1 -> Terminator/1
  Anti-windup AoA/1 -> Terminator1/1

== system F16ASYM_Controlled_AoA/Primary Controller/PI Primary Controller/Longitudinal Controller: AoA or A_w_z/Longitudinal controller in AoA ==
  A_w_z des : Inport
  AoA des (rad) : Inport  Port=2
  Anti-windup A_w_z : Inport  Port=3
  Anti-windup AoA : Inport  Port=4
  All meas : Inport  Port=5
  Bus Selector : BusSelector  OutputSignals=signal1.AoA meas (rad)
  PI Controller: Aoa  controller : Adaptive_FaultTolerantControl/PI Controller  delta=0  K_a=0  y_i=trim_state(8)  Des_way=auto  omega_n=3  xi=0.9  Z1=-50  K_b=5  f_i=0.1  f_c=1
  Terminator : Terminator
  Terminator1 : Terminator
  alpha_dot_c : Outport
  wires:
  Anti-windup AoA/1 -> PI Controller: Aoa  controller/3
  Anti-windup A_w_z/1 -> Terminator1/1
  A_w_z des/1 -> Terminator/1
  AoA des (rad)/1 -> PI Controller: Aoa  controller/1
  Bus Selector/1 -> PI Controller: Aoa  controller/2  "<AoA meas (rad)>"
  PI Controller: Aoa  controller/1 -> alpha_dot_c/1
  All meas/1 -> Bus Selector/1

== system F16ASYM_Controlled_AoA/Primary Controller/P  + Crossed NN + AWU+Lim + hand-over/P controller + adaptive Crossed NN + AWU+Lim    in ACC /Long Dyn Inversion: alpha_dot ->q/Completed ==
  alpha_dot_c : Inport
  All_meas : Inport  Port=2
  A_w_z : Selector  InputPortWidth=3  IndexOptions=Index vector (dialog)  Indices=3  OutputSizes=1
  Add : Sum
  Bus Selector : BusSelector  OutputSignals=signal1.AoA meas (rad),signal1.omega_b meas (rad/s),signal1.SS meas (rad),signal1.V_TAS (m/s),signal2.A_w_CG
  Display : Display
  Display1 : Display
  Display2 : Display
  Divide{,1..3} (4 alike) : Product  Inputs=**
  Divide4 : Product  Inputs=/*
  Selector : Selector  InputPortWidth=3  IndexOptions=Index vector (dialog)  Indices=1  OutputSizes=1
  Selector1 : Selector  InputPortWidth=3  IndexOptions=Index vector (dialog)  Indices=3  OutputSizes=1
  Trigonometric Function : Trigonometry  Operator=sincos
  Trigonometric Function1 : Trigonometry  Operator=tan
  Trigonometric Function2 : Trigonometry  Operator=cos
  "q_c " : Sum  Inputs=++-
  q_c : Outport
  wires:
  Trigonometric Function/1 -> Divide1/1
  Bus Selector/1 -> Trigonometric Function/1  "<AoA meas (rad)>"
  Selector/1 -> Divide/2
  Bus Selector/2 -> Selector1/1, Selector/1  "<omega_b meas (rad/s)>"
  Divide2/1 -> "q_c "/2, Display1/1
  Selector1/1 -> Divide1/2
  Divide3/1 -> Divide4/1
  alpha_dot_c/1 -> "q_c "/1, Display/1
  All_meas/1 -> Bus Selector/1
  Bus Selector/5 -> A_w_z/1  "<A_w_CG>"
  Bus Selector/3 -> Trigonometric Function1/1, Trigonometric Function2/1  "<SS meas (rad)>"
  Divide4/1 -> "q_c "/3
  "q_c "/1 -> q_c/1
  Divide/1 -> Add/1
  Bus Selector/4 -> Divide3/2  "<V_TAS (m/s)>"
  Add/1 -> Divide2/1
  Trigonometric Function1/1 -> Divide2/2
  Divide1/1 -> Add/2
  Trigonometric Function2/1 -> Divide3/1
  Trigonometric Function/2 -> Divide/1
  A_w_z/1 -> Display2/1, Divide4/2

== system F16ASYM_Controlled_AoA/Primary Controller/P  + Crossed NN + AWU+Lim + hand-over/P controller + adaptive Crossed NN + AWU+Lim    in ACC /Long Dyn Inversion: alpha_dot ->q/Simplified ==
  alpha_dot_c : Inport
  All_meas : Inport  Port=2
  A_b_z : Selector  InputPortWidth=3  IndexOptions=Index vector (dialog)  Indices=3  OutputSizes=1
  Bus Selector : BusSelector  OutputSignals=signal2.A_b_CG,signal1.V_TAS (m/s)
  Display : Display
  Divide4 : Product  Inputs=*/
  "q_c " : Sum  Inputs=+-
  q_c : Outport
  wires:
  "q_c "/1 -> q_c/1
  All_meas/1 -> Bus Selector/1
  alpha_dot_c/1 -> "q_c "/1, Display/1
  Bus Selector/2 -> Divide4/2  "<V_TAS (m/s)>"
  Divide4/1 -> "q_c "/2
  A_b_z/1 -> Divide4/1  "A_b_z"
  Bus Selector/1 -> A_b_z/1  "<A_b_CG>"

== system F16ASYM_Controlled_AoA/Primary Controller/P  + Crossed NN + AWU+Lim + hand-over/P controller + adaptive Crossed NN + AWU+Lim    in ACC /Longitudinal controller in A_w_z/Accel rate --> AoA rate! ==
  All_meas : Inport
  1/a_1 : Gain  Gain=1/a1
  Bus Selector : BusSelector  OutputSignals=signal2.q (Pa)
  Divide : Product  Inputs=**
  Divide2 : Product  Inputs=*/
  S : Constant  Value=27.87
  mass : Constant  Value=9295.44
  A_w  to AoA rates factor : Outport
  wires:
  S/1 -> Divide/1
  Bus Selector/1 -> Divide/2  "<q (Pa)>"
  mass/1 -> Divide2/1
  Divide/1 -> Divide2/2
  Divide2/1 -> 1/a_1/1
  All_meas/1 -> Bus Selector/1
  1/a_1/1 -> A_w  to AoA rates factor/1

== system F16ASYM_Controlled_AoA/Primary Controller/P  + Crossed NN + AWU+Lim + hand-over/P controller + adaptive Crossed NN + AWU+Lim    in ACC /Longitudinal controller in A_w_z/Stall protection ==
  alpha_dot des : Inport
  All meas : Inport  Port=2
  Bus Selector : BusSelector  OutputSignals=signal1.AoA meas (rad)
  MATLAB Function : MATLAB Function  TreatAsAtomicUnit=on
  AoA des : Outport
  wires:
  alpha_dot des/1 -> MATLAB Function/1(alpha_dot)
  MATLAB Function/1(alpha_dot_out) -> AoA des/1
  All meas/1 -> Bus Selector/1
  Bus Selector/1 -> MATLAB Function/2(alpha)  "<AoA meas (rad)>"

== system F16ASYM_Controlled_AoA/Primary Controller/P  + Crossed NN + AWU+Lim + hand-over/P controller + adaptive Crossed NN + AWU+Lim    in ACC /Physical limitation/Moments ==
  C_L : Inport
  C_M : Inport  Port=2
  C_N : Inport  Port=3
  q : Inport  Port=4
  B span : Constant  Value=9.144
  CMA : Constant  Value=3.45
  Divide : Product  Inputs=**
  Divide1 : Product  Inputs=***
  Divide2 : Product  Inputs=**
  Divide3 : Product  Inputs=***
  Divide4 : Product  Inputs=**
  S_w : Constant  Value=27.87
  S_w1 : Constant  Value=27.87
  q1 : InportShadow  Port=4
  L : Outport
  M : Outport  Port=2
  N : Outport  Port=3
  wires:
  Divide4/1 -> M/1  "M"
  Divide3/1 -> Divide4/2
  C_M/1 -> Divide4/1
  CMA/1 -> Divide3/3
  S_w1/1 -> Divide3/2
  q1/1 -> Divide3/1
  Divide2/1 -> N/1  "N"
  C_N/1 -> Divide2/2
  Divide/1 -> L/1  "L"
  Divide1/1 -> Divide/2, Divide2/1
  C_L/1 -> Divide/1
  B span/1 -> Divide1/3
  S_w/1 -> Divide1/2
  q/1 -> Divide1/1

== system F16ASYM_Controlled_AoA/Primary Controller/P  + Crossed NN + AWU+Lim + hand-over/P controller + adaptive Crossed NN + AWU+Lim   in AoA/Long Dyn Inversion: alpha_dot ->q/Completed ==
  alpha_dot_c : Inport
  All_meas : Inport  Port=2
  A_w_z : Selector  InputPortWidth=3  IndexOptions=Index vector (dialog)  Indices=3  OutputSizes=1
  Add : Sum
  Bus Selector : BusSelector  OutputSignals=signal1.AoA meas (rad),signal1.omega_b meas (rad/s),signal1.SS meas (rad),signal1.V_TAS (m/s),signal2.A_w_CG
  Display : Display
  Display1 : Display
  Display2 : Display
  Divide{,1..3} (4 alike) : Product  Inputs=**
  Divide4 : Product  Inputs=/*
  Selector : Selector  InputPortWidth=3  IndexOptions=Index vector (dialog)  Indices=1  OutputSizes=1
  Selector1 : Selector  InputPortWidth=3  IndexOptions=Index vector (dialog)  Indices=3  OutputSizes=1
  Trigonometric Function : Trigonometry  Operator=sincos
  Trigonometric Function1 : Trigonometry  Operator=tan
  Trigonometric Function2 : Trigonometry  Operator=cos
  "q_c " : Sum  Inputs=++-
  q_c : Outport
  wires:
  Trigonometric Function/1 -> Divide1/1
  Bus Selector/1 -> Trigonometric Function/1  "<AoA meas (rad)>"
  Selector/1 -> Divide/2
  Bus Selector/2 -> Selector1/1, Selector/1  "<omega_b meas (rad/s)>"
  Divide2/1 -> "q_c "/2, Display1/1
  Selector1/1 -> Divide1/2
  Divide3/1 -> Divide4/1
  alpha_dot_c/1 -> "q_c "/1, Display/1
  All_meas/1 -> Bus Selector/1
  Bus Selector/5 -> A_w_z/1  "<A_w_CG>"
  Bus Selector/3 -> Trigonometric Function1/1, Trigonometric Function2/1  "<SS meas (rad)>"
  Divide4/1 -> "q_c "/3
  "q_c "/1 -> q_c/1
  Divide/1 -> Add/1
  Bus Selector/4 -> Divide3/2  "<V_TAS (m/s)>"
  Add/1 -> Divide2/1
  Trigonometric Function1/1 -> Divide2/2
  Divide1/1 -> Add/2
  Trigonometric Function2/1 -> Divide3/1
  Trigonometric Function/2 -> Divide/1
  A_w_z/1 -> Display2/1, Divide4/2

== system F16ASYM_Controlled_AoA/Primary Controller/P  + Crossed NN + AWU+Lim + hand-over/P controller + adaptive Crossed NN + AWU+Lim   in AoA/Long Dyn Inversion: alpha_dot ->q/Simplified ==
  alpha_dot_c : Inport
  All_meas : Inport  Port=2
  A_b_z : Selector  InputPortWidth=3  IndexOptions=Index vector (dialog)  Indices=3  OutputSizes=1
  Bus Selector : BusSelector  OutputSignals=signal2.A_b_CG,signal1.V_TAS (m/s)
  Display : Display
  Divide4 : Product  Inputs=*/
  "q_c " : Sum  Inputs=+-
  q_c : Outport
  wires:
  "q_c "/1 -> q_c/1
  All_meas/1 -> Bus Selector/1
  alpha_dot_c/1 -> "q_c "/1, Display/1
  Bus Selector/2 -> Divide4/2  "<V_TAS (m/s)>"
  Divide4/1 -> "q_c "/2
  A_b_z/1 -> Divide4/1  "A_b_z"
  Bus Selector/1 -> A_b_z/1  "<A_b_CG>"

== system F16ASYM_Controlled_AoA/Primary Controller/P  + Crossed NN + AWU+Lim + hand-over/P controller + adaptive Crossed NN + AWU+Lim   in AoA/Physical limitation/Moments ==
  C_L : Inport
  C_M : Inport  Port=2
  C_N : Inport  Port=3
  q : Inport  Port=4
  B span : Constant  Value=9.144
  CMA : Constant  Value=3.45
  Divide : Product  Inputs=**
  Divide1 : Product  Inputs=***
  Divide2 : Product  Inputs=**
  Divide3 : Product  Inputs=***
  Divide4 : Product  Inputs=**
  S_w : Constant  Value=27.87
  S_w1 : Constant  Value=27.87
  q1 : InportShadow  Port=4
  L : Outport
  M : Outport  Port=2
  N : Outport  Port=3
  wires:
  Divide4/1 -> M/1  "M"
  Divide3/1 -> Divide4/2
  C_M/1 -> Divide4/1
  CMA/1 -> Divide3/3
  S_w1/1 -> Divide3/2
  q1/1 -> Divide3/1
  Divide2/1 -> N/1  "N"
  C_N/1 -> Divide2/2
  Divide/1 -> L/1  "L"
  Divide1/1 -> Divide/2, Divide2/1
  C_L/1 -> Divide/1
  B span/1 -> Divide1/3
  S_w/1 -> Divide1/2
  q/1 -> Divide1/1

== system F16ASYM_Controlled_AoA/Primary Controller/P controller/Longitudinal Controller: AoA or A_w_z/Longitudinal controller in A_w_z/Accel rate --> AoA rate! ==
  A_w_z dot : Inport
  All_meas : Inport  Port=2
  1/a_1 : Gain  Gain=1/a1
  Bus Selector : BusSelector  OutputSignals=signal2.q (Pa)
  Divide : Product  Inputs=**
  Divide1 : Product  Inputs=**
  Divide2 : Product  Inputs=*/
  S : Constant  Value=27.87
  mass : Constant  Value=9295.44
  alpha_dot des : Outport
  wires:
  1/a_1/1 -> alpha_dot des/1  "ALPHA_DOT"
  All_meas/1 -> Bus Selector/1
  Divide2/1 -> 1/a_1/1
  Divide/1 -> Divide2/2
  Divide1/1 -> Divide2/1
  mass/1 -> Divide1/2
  Bus Selector/1 -> Divide/2  "<q (Pa)>"
  S/1 -> Divide/1
  A_w_z dot/1 -> Divide1/1

== system F16ASYM_Controlled_AoA/Primary Controller/P controller + adaptive Crossed NN/Longitudinal Controller: AoA or A_w_z/Longitudinal controller in A_w_z/Accel rate --> AoA rate! ==
  All_meas : Inport
  1/a_1 : Gain  Gain=1/a1
  Bus Selector : BusSelector  OutputSignals=signal2.q (Pa)
  Divide : Product  Inputs=**
  Divide2 : Product  Inputs=*/
  S : Constant  Value=27.87
  mass : Constant  Value=9295.44
  A_w  to AoA rates factor : Outport
  wires:
  1/a_1/1 -> A_w  to AoA rates factor/1
  All_meas/1 -> Bus Selector/1
  Divide2/1 -> 1/a_1/1
  Divide/1 -> Divide2/2
  mass/1 -> Divide2/1
  Bus Selector/1 -> Divide/2  "<q (Pa)>"
  S/1 -> Divide/1

== system F16ASYM_Controlled_AoA/Primary Controller/P controller + adaptive Crossed NN + AWU+Lim /Longitudinal Controller: AoA or A_w_z/Longitudinal controller in A_w_z/Accel rate --> AoA rate! ==
  All_meas : Inport
  1/a_1 : Gain  Gain=1/a1
  Bus Selector : BusSelector  OutputSignals=signal2.q (Pa)
  Divide : Product  Inputs=**
  Divide2 : Product  Inputs=*/
  S : Constant  Value=27.87
  mass : Constant  Value=9295.44
  A_w  to AoA rates factor : Outport
  wires:
  S/1 -> Divide/1
  Bus Selector/1 -> Divide/2  "<q (Pa)>"
  mass/1 -> Divide2/1
  Divide/1 -> Divide2/2
  Divide2/1 -> 1/a_1/1
  All_meas/1 -> Bus Selector/1
  1/a_1/1 -> A_w  to AoA rates factor/1

== system F16ASYM_Controlled_AoA/Primary Controller/P controller + adaptive Crossed NN + AWU+Lim /Longitudinal Controller: AoA or A_w_z/Longitudinal controller in A_w_z/Stall protection ==
  alpha_dot des : Inport
  All meas : Inport  Port=2
  Bus Selector : BusSelector  OutputSignals=signal1.AoA meas (rad)
  MATLAB Function : MATLAB Function  TreatAsAtomicUnit=on
  AoA des : Outport
  wires:
  alpha_dot des/1 -> MATLAB Function/1(alpha_dot)
  MATLAB Function/1(alpha_dot_out) -> AoA des/1
  All meas/1 -> Bus Selector/1
  Bus Selector/1 -> MATLAB Function/2(alpha)  "<AoA meas (rad)>"

== system F16ASYM_Controlled_AoA/Primary Controller/P controller + adaptive Isolated NN/Longitudinal Controller: AoA or A_w_z/Longitudinal controller in A_w_z/Accel rate --> AoA rate! ==
  All_meas : Inport
  1/a_1 : Gain  Gain=1/a1
  Bus Selector : BusSelector  OutputSignals=signal2.q (Pa)
  Divide : Product  Inputs=**
  Divide2 : Product  Inputs=*/
  S : Constant  Value=27.87
  mass : Constant  Value=9295.44
  A_w  to AoA rates factor : Outport
  wires:
  S/1 -> Divide/1
  Bus Selector/1 -> Divide/2  "<q (Pa)>"
  mass/1 -> Divide2/1
  Divide/1 -> Divide2/2
  Divide2/1 -> 1/a_1/1
  All_meas/1 -> Bus Selector/1
  1/a_1/1 -> A_w  to AoA rates factor/1
